simulink model "engine_control_codegen"  (R2024a)
settings: Solver=FixedStepDiscrete  StartTime=0.0  StopTime=10.0  FixedStep=0.01  RelTol=1e-3
model workspace (MAT data in the model file):
  DD = Simulink.Parameter
  DD.Value = 3
  DD.Complexity = 'real'
  DD.Dimensions = [1 1]
  DD.DataType = 'uint8'
  NN = Simulink.Parameter
  NN.Value = 2
  NN.Complexity = 'real'
  NN.Dimensions = [1 1]
  NN.DataType = 'uint8'
  PP = Simulink.Parameter
  PP.Value = 0
  PP.Complexity = 'real'
  PP.Dimensions = [1 1]
  PP.DataType = 'uint8'
  RR = Simulink.Parameter
  RR.Value = 1
  RR.Complexity = 'real'
  RR.Dimensions = [1 1]
  RR.DataType = 'uint8'
settings Model: Creator=18283  LastModifiedBy=18283
settings OptimizationCC: EnhancedBackFolding=on  PassReuseOutputArgsAs=Individual arguments  ZeroExternalMemoryAtStartup=off  ZeroInternalMemoryAtStartup=off  OptimizeBlockOrder=speed  DifferentSizesBufferReuse=on  OptimizationCustomize=off  EfficientTunableParamExpr=on
settings DebuggingCC: ParameterTunabilityLossMsg=error
settings SFSimCC: MATLABDynamicMemAlloc=off
settings RTWCC: Description=Embedded Coder  SystemTargetFile=ert.tlc  TemplateMakefile=ert_default_tmf
settings CodeAppCC: ForceParamTrailComments=on  IgnoreCustomStorageClasses=off  OperatorAnnotations=on  SimulinkDataObjDesc=on  SFDataObjDesc=on  InsertBlockDesc=on
settings ERTTargetCC: TargetLangStandard=C99 (ISO)  GenerateSampleERTMain=on  ERTCustomFileTemplate=example_file_process.tlc

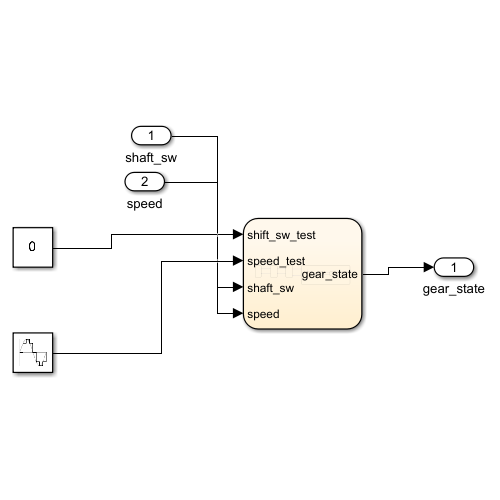
[thumbnail: Simulink's stored preview of the top-level diagram]
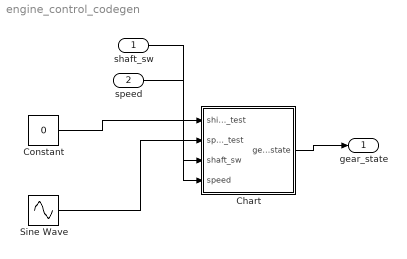
== system engine_control_codegen ==
  shaft_sw : Inport  OutDataTypeStr=uint8  SampleTime=0.01
  speed : Inport  Port=2  OutDataTypeStr=single  SampleTime=0.01
  Chart : Stateflow chart  TreatAsAtomicUnit=on
  Constant : Constant  Value=0
  Sine Wave : Sin  Amplitude=100  SampleTime=0.01
  gear_state : Outport
  wires:
  Constant/1 -> Chart/1(shift_sw_test)
  Sine Wave/1 -> Chart/2(speed_test)
  shaft_sw/1 -> Chart/3(shaft_sw)
  speed/1 -> Chart/4(speed)
  Chart/1(gear_state) -> gear_state/1

== stateflow chart engine_control_codegen/Chart ==
  state P
    entry: gear_state=PP;
  state R
    entry: gear_state=RR;
  state N
    entry: gear_state=NN;
  state D
    entry: gear_state=DD;
    state D1
    state D2
    state D3
    state D4
    (default) -> D1
    D3 -> D4 [order 1] : [speed>60]
    D1 -> D2 : [speed>20]
    D2 -> D3 [order 1] : [speed>40]
    D4 -> D3 : [speed<55]
    D3 -> D2 [order 2] : [speed<35]
    D2 -> D1 [order 2] : [speed<15]
  (default) -> P
  R -> N [order 1] : [shaft_sw==NN]
  P -> R : [shaft_sw==RR]
  N -> D [order 1] : [shaft_sw==DD]
  R -> P [order 2] : [shaft_sw==PP]
  N -> R [order 2] : [shaft_sw==RR]
  D -> N : [shaft_sw==NN]
  data: shift_sw_test input; speed_test input; PP parameter uint8 size=1; RR parameter uint8 size=1; NN parameter uint8 size=1; DD parameter uint8 size=1; shaft_sw input uint8 size=1; speed input single size=1; gear_state output uint8 size=1
